simulink model "MD_sfunc_test_6dof"  (R2024a)
settings: Solver=FixedStepDiscrete  StartTime=0.0  StopTime=TMax  FixedStep=dt  RelTol=1e-3
PreLoadFcn:
  | initializeSimulation
  | initializeSCRAMNetGT
settings Model: Creator=mvetsch  LastModifiedBy=mcdevin
settings SolverCC: AlgebraicLoopSolver=TrustRegion
settings DataIOCC: SaveFormat=Array  SaveOutput=off  SignalLogging=off  SaveTime=off  ReturnWorkspaceOutputs=off  SignalLoggingName=sigsOut
settings OptimizationCC: BlockReduction=off  OptimizeBlockIOStorage=off  BufferReuse=off  GlobalBufferReuse=off  ExpressionFolding=off  ExpressionDepthLimit=2147483647  LocalBlockOutputs=off  InitFltsAndDblsToZero=on  EfficientFloat2IntCast=on  LifeSpan=inf  SimCompilerOptimization=on  OptimizeDataStoreBuffers=off  BusAssignmentInplaceUpdate=off
settings DebuggingCC: SaveWithParameterizedLinksMsg=none  CheckSSInitialOutputMsg=off  UnderspecifiedInitializationDetection=Classic  MergeDetectMultiDrivingBlocksExec=none  UnconnectedInputMsg=warning  UnconnectedOutputMsg=warning  UnconnectedLineMsg=warning  AllowSymbolicDim=off  StateNameClashWarn=warning  PregeneratedLibrarySubsystemCodeDiagnostic=none  SFUnexpectedBacktrackingDiag=warning  SFNoUnconditionalDefaultTransitionDiag=warning  SFExecutionAtInitializationDiag=none  ArithmeticOperatorsInVariantConditions=warning
settings HardwareCC: ProdBitPerPointer=32  ProdBitPerSizeT=32  ProdBitPerPtrDiffT=32  ProdLargestAtomicFloat=None  ProdWordSize=32  ProdLongLongMode=on  ProdHWDeviceType=Generic->32-bit x86 compatible  TargetHWDeviceType=32-bit Generic
settings ModelReferenceCC: EnableRefExpFcnMdlSchedulingChecks=on  PropagateSignalLabelsOutOfModel=off
settings SFSimCC: SimCustomHeaderCode="#include \"PredictorCorrector.h\""  SimUserSources=PredictorCorrector.c  SimUserIncludeDirs="\"C:\\Program Files\\OpenFresco\\SourceCode\\SRC\\experimentalControl\\Simulink\\HybridSimToolbox\""  SimUseLocalCustomCode=off  SimParseCustomCode=off  CustomCodeUndefinedFunction=UseInterfaceOnly
settings RTWCC: Description=Simulink Real-Time  SystemTargetFile=slrt.tlc  TemplateMakefile=slrt_default_tmf  RTWUseLocalCustomCode=off  CustomHeaderCode="#include \"PredictorCorrector.h\""  CustomSource=PredictorCorrector.c  RTWCompilerOptimization=on  GPUComputeCapability=3.5
settings RTWCC: CustomInclude=|
  | "C:\Program Files\OpenFresco\SourceCode\SRC\experimentalControl\Simulink\HybridSimToolbox"
  | "C:\Projects\Michael\openfast\build\bin"
settings CodeAppCC: StateflowObjectComments=on
settings SimulinkRealTimeCC: TargetFcnLib=ansi_tfl_tmw.mat  InstructionSetFMA=off  OptimizeReductions=off  LogToMDFFile=off
settings ConfigComp: CovMetricSettings=dw  CovSaveCumulativeToWorkspaceVar=on  CovSaveSingleToWorkspaceVar=on  CovExternalEMLEnable=off

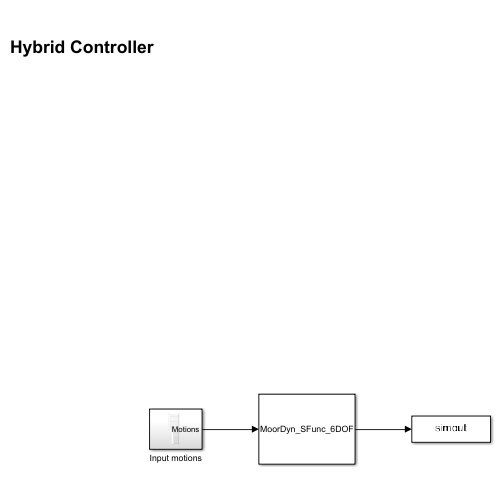
[thumbnail: Simulink's stored preview of the top-level diagram]
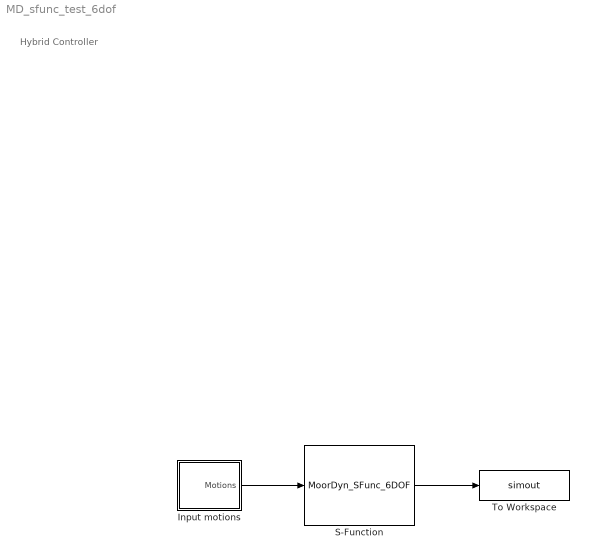
== system MD_sfunc_test_6dof ==
  note: Hybrid Controller
  Input motions : Subsystem
  S-Function : S-Function  FunctionName=MoorDyn_SFunc_6DOF  Parameters=MD_InputFileName, dt, TMax  SFunctionDeploymentMode=off  EnableBusSupport=off
  To Workspace : ToWorkspace  VariableName=simout  SaveFormat=Timeseries  SampleTime=-1
  wires:
  S-Function/1 -> To Workspace/1
  Input motions/1(Motions) -> S-Function/1

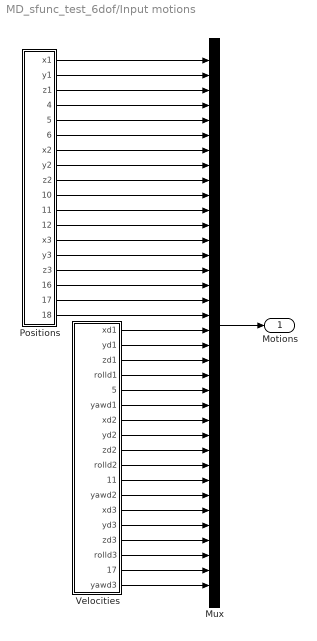
== system MD_sfunc_test_6dof/Input motions ==
  Mux : Mux  Inputs=36
  Positions : Subsystem
  Velocities : Subsystem
  Motions : Outport  VectorParamsAs1DForOutWhenUnconnected=off
  wires:
  Mux/1 -> Motions/1
  Positions/17(pitch3) -> Mux/17
  Positions/16(roll3) -> Mux/16
  Positions/15(z3) -> Mux/15
  Positions/14(y3) -> Mux/14
  Positions/13(x3) -> Mux/13
  Positions/12(yaw2) -> Mux/12
  Positions/11(pitch2) -> Mux/11
  Positions/10(roll2) -> Mux/10
  Positions/9(z2) -> Mux/9
  Positions/8(y2) -> Mux/8
  Positions/7(x2) -> Mux/7
  Positions/6(yaw1) -> Mux/6
  Positions/5(pitch1) -> Mux/5
  Positions/4(roll1) -> Mux/4
  Positions/3(z1) -> Mux/3
  Positions/2(y1) -> Mux/2
  Positions/1(x1) -> Mux/1
  Positions/18(yaw3) -> Mux/18
  Velocities/1(xd1) -> Mux/19
  Velocities/2(yd1) -> Mux/20
  Velocities/3(zd1) -> Mux/21
  Velocities/5(pitchd1) -> Mux/23
  Velocities/4(rolld1) -> Mux/22
  Velocities/6(yawd1) -> Mux/24
  Velocities/7(xd2) -> Mux/25
  Velocities/8(yd2) -> Mux/26
  Velocities/9(zd2) -> Mux/27
  Velocities/10(rolld2) -> Mux/28
  Velocities/11(pitchd2) -> Mux/29
  Velocities/12(yawd2) -> Mux/30
  Velocities/13(xd3) -> Mux/31
  Velocities/14(yd3) -> Mux/32
  Velocities/15(zd3) -> Mux/33
  Velocities/16(rolld3) -> Mux/34
  Velocities/17(pitchd3) -> Mux/35
  Velocities/18(yawd3) -> Mux/36

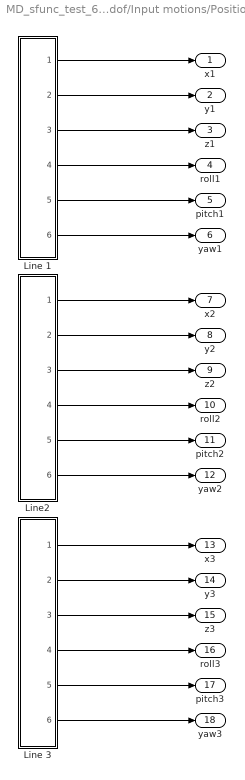
== system MD_sfunc_test_6dof/Input motions/Positions ==
  Line 1 : Subsystem
  Line 3 : Subsystem
  Line2 : Subsystem
  x1 : Outport
  y1 : Outport  Port=2
  z1 : Outport  Port=3
  roll1 : Outport  Port=4
  pitch1 : Outport  Port=5
  yaw1 : Outport  Port=6
  x2 : Outport  Port=7
  y2 : Outport  Port=8
  z2 : Outport  Port=9
  roll2 : Outport  Port=10
  pitch2 : Outport  Port=11
  yaw2 : Outport  Port=12
  x3 : Outport  Port=13
  y3 : Outport  Port=14
  z3 : Outport  Port=15
  roll3 : Outport  Port=16
  pitch3 : Outport  Port=17
  yaw3 : Outport  Port=18
  wires:
  Line 3/1(Out1) -> x3/1
  Line 3/2(Out2) -> y3/1
  Line 3/3(Out3) -> z3/1
  Line 3/4(Out4) -> roll3/1
  Line 3/5(Out5) -> pitch3/1
  Line 3/6(Out6) -> yaw3/1
  Line2/1(Out1) -> x2/1
  Line2/2(Out2) -> y2/1
  Line2/3(Out3) -> z2/1
  Line2/4(Out4) -> roll2/1
  Line2/5(Out5) -> pitch2/1
  Line2/6(Out6) -> yaw2/1
  Line 1/1(Out1) -> x1/1
  Line 1/2(Out2) -> y1/1
  Line 1/3(Out3) -> z1/1
  Line 1/4(Out4) -> roll1/1
  Line 1/5(Out5) -> pitch1/1
  Line 1/6(Out6) -> yaw1/1

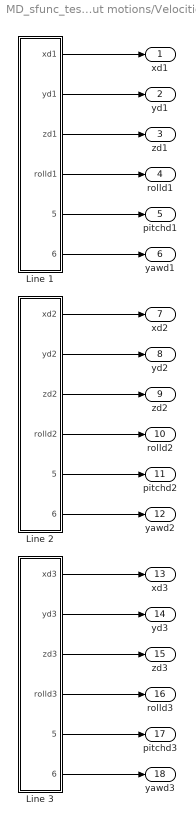
== system MD_sfunc_test_6dof/Input motions/Velocities ==
  Line 1 : Subsystem
  Line 2 : Subsystem
  Line 3 : Subsystem
  xd1 : Outport
  yd1 : Outport  Port=2
  zd1 : Outport  Port=3
  rolld1 : Outport  Port=4
  pitchd1 : Outport  Port=5
  yawd1 : Outport  Port=6
  xd2 : Outport  Port=7
  yd2 : Outport  Port=8
  zd2 : Outport  Port=9
  rolld2 : Outport  Port=10
  pitchd2 : Outport  Port=11
  yawd2 : Outport  Port=12
  xd3 : Outport  Port=13
  yd3 : Outport  Port=14
  zd3 : Outport  Port=15
  rolld3 : Outport  Port=16
  pitchd3 : Outport  Port=17
  yawd3 : Outport  Port=18
  wires:
  Line 1/1(xd1) -> xd1/1
  Line 1/2(yd1) -> yd1/1
  Line 1/3(zd1) -> zd1/1
  Line 1/4(rolld1) -> rolld1/1
  Line 1/5(pitchd1) -> pitchd1/1
  Line 1/6(yawd1) -> yawd1/1
  Line 2/4(rolld2) -> rolld2/1
  Line 2/2(yd2) -> yd2/1
  Line 2/6(yawd2) -> yawd2/1
  Line 2/1(xd2) -> xd2/1
  Line 2/5(pitchd2) -> pitchd2/1
  Line 2/3(zd2) -> zd2/1
  Line 3/4(rolld3) -> rolld3/1
  Line 3/2(yd3) -> yd3/1
  Line 3/6(yawd3) -> yawd3/1
  Line 3/1(xd3) -> xd3/1
  Line 3/5(pitchd3) -> pitchd3/1
  Line 3/3(zd3) -> zd3/1

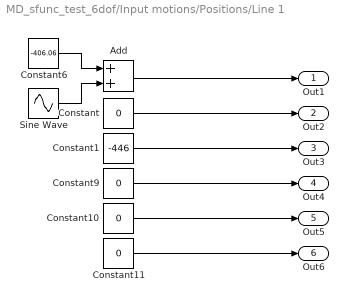
== system MD_sfunc_test_6dof/Input motions/Positions/Line 1 ==
  Add : Sum
  Constant{,9..11} (4 alike) : Constant  Value=0
  Constant1 : Constant  Value=-446
  Constant6 : Constant  Value=-406.06
  Sine Wave : Sin  Amplitude=5  Frequency=0.314159265358979323846  SampleTime=0
  Out1 : Outport
  Out2 : Outport  Port=2
  Out3 : Outport  Port=3
  Out4 : Outport  Port=4
  Out5 : Outport  Port=5
  Out6 : Outport  Port=6
  wires:
  Sine Wave/1 -> Add/2
  Constant6/1 -> Add/1
  Add/1 -> Out1/1
  Constant11/1 -> Out6/1
  Constant1/1 -> Out3/1
  Constant/1 -> Out2/1
  Constant10/1 -> Out5/1
  Constant9/1 -> Out4/1

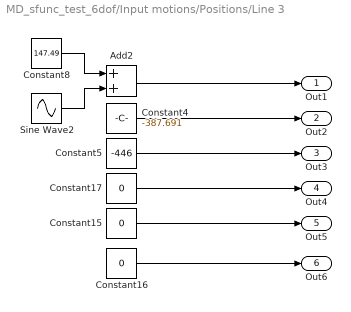
== system MD_sfunc_test_6dof/Input motions/Positions/Line 3 ==
  Add2 : Sum
  Constant15 : Constant  Value=0
  Constant16 : Constant  Value=0
  Constant17 : Constant  Value=0
  Constant4 : Constant  Value=-387.691
  Constant5 : Constant  Value=-446
  Constant8 : Constant  Value=147.49
  Sine Wave2 : Sin  Amplitude=5  Frequency=0.314159265358979323846  SampleTime=0
  Out1 : Outport
  Out2 : Outport  Port=2
  Out3 : Outport  Port=3
  Out4 : Outport  Port=4
  Out5 : Outport  Port=5
  Out6 : Outport  Port=6
  wires:
  Constant15/1 -> Out5/1
  Constant8/1 -> Add2/1
  Constant5/1 -> Out3/1
  Constant17/1 -> Out4/1
  Constant16/1 -> Out6/1
  Sine Wave2/1 -> Add2/2
  Add2/1 -> Out1/1
  Constant4/1 -> Out2/1

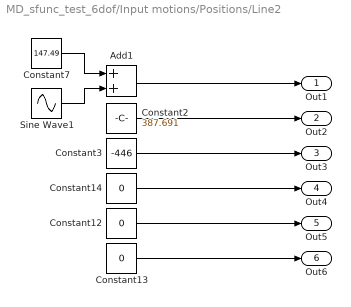
== system MD_sfunc_test_6dof/Input motions/Positions/Line2 ==
  Add1 : Sum
  Constant12 : Constant  Value=0
  Constant13 : Constant  Value=0
  Constant14 : Constant  Value=0
  Constant2 : Constant  Value=387.691
  Constant3 : Constant  Value=-446
  Constant7 : Constant  Value=147.49
  Sine Wave1 : Sin  Amplitude=5  Frequency=0.314159265358979323846  SampleTime=0
  Out1 : Outport
  Out2 : Outport  Port=2
  Out3 : Outport  Port=3
  Out4 : Outport  Port=4
  Out5 : Outport  Port=5
  Out6 : Outport  Port=6
  wires:
  Add1/1 -> Out1/1
  Sine Wave1/1 -> Add1/2
  Constant3/1 -> Out3/1
  Constant7/1 -> Add1/1
  Constant12/1 -> Out5/1
  Constant2/1 -> Out2/1
  Constant13/1 -> Out6/1
  Constant14/1 -> Out4/1

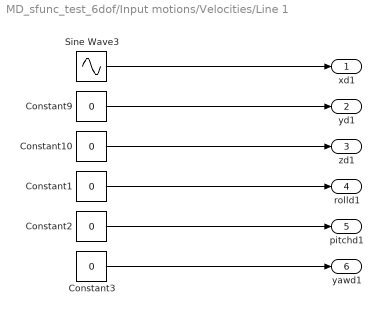
== system MD_sfunc_test_6dof/Input motions/Velocities/Line 1 ==
  Constant{1..3,9..10} (5 alike) : Constant  Value=0
  Sine Wave3 : Sin  Amplitude=0.314159265358979323846  Frequency=0.314159265358979323846  Phase=3.14159265358979323846 / 2  SampleTime=0
  xd1 : Outport
  yd1 : Outport  Port=2
  zd1 : Outport  Port=3
  rolld1 : Outport  Port=4
  pitchd1 : Outport  Port=5
  yawd1 : Outport  Port=6
  wires:
  Constant1/1 -> rolld1/1
  Constant2/1 -> pitchd1/1
  Sine Wave3/1 -> xd1/1
  Constant9/1 -> yd1/1
  Constant10/1 -> zd1/1
  Constant3/1 -> yawd1/1

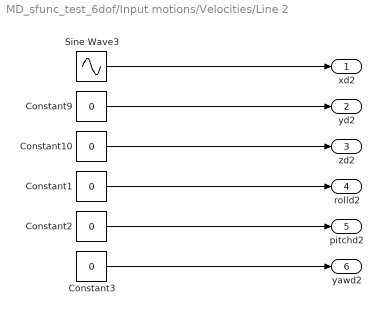
== system MD_sfunc_test_6dof/Input motions/Velocities/Line 2 ==
  Constant{1..3,9..10} (5 alike) : Constant  Value=0
  Sine Wave3 : Sin  Amplitude=0.314159265358979323846  Frequency=0.314159265358979323846  Phase=3.14159265358979323846 / 2  SampleTime=0
  xd2 : Outport
  yd2 : Outport  Port=2
  zd2 : Outport  Port=3
  rolld2 : Outport  Port=4
  pitchd2 : Outport  Port=5
  yawd2 : Outport  Port=6
  wires:
  Constant1/1 -> rolld2/1
  Constant2/1 -> pitchd2/1
  Sine Wave3/1 -> xd2/1
  Constant9/1 -> yd2/1
  Constant10/1 -> zd2/1
  Constant3/1 -> yawd2/1

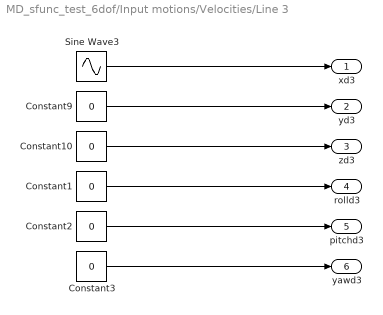
== system MD_sfunc_test_6dof/Input motions/Velocities/Line 3 ==
  Constant{1..3,9..10} (5 alike) : Constant  Value=0
  Sine Wave3 : Sin  Amplitude=0.314159265358979323846  Frequency=0.314159265358979323846  Phase=3.14159265358979323846 / 2  SampleTime=0
  xd3 : Outport
  yd3 : Outport  Port=2
  zd3 : Outport  Port=3
  rolld3 : Outport  Port=4
  pitchd3 : Outport  Port=5
  yawd3 : Outport  Port=6
  wires:
  Constant1/1 -> rolld3/1
  Constant2/1 -> pitchd3/1
  Sine Wave3/1 -> xd3/1
  Constant9/1 -> yd3/1
  Constant10/1 -> zd3/1
  Constant3/1 -> yawd3/1
